simulink model "Esercizio2"  (R2020a)
settings: Solver=VariableStepAuto  StartTime=0.0  StopTime=100  RelTol=1e-3
values from neighbouring files (symbols this model uses):
  D = 0.05    [parameters.m]
  g = 9.8    [parameters.m]
  K = 5    [parameters.m]
  M = 1    [parameters.m]
  x_0 = 10    [parameters.m]
settings Model: Creator=bogda  LastModifiedBy=bogda

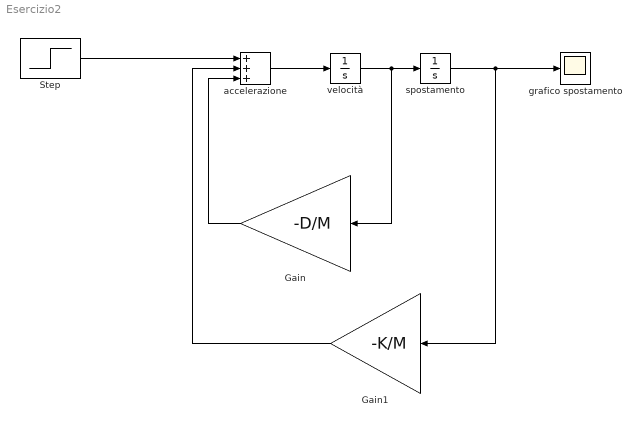
== system Esercizio2 ==
  Gain : Gain  Gain=-D/M
  Gain1 : Gain  Gain=-K/M
  Step : Step  After=g  SampleTime=0
  accelerazione : Sum  Inputs=+++
  grafico spostamento : Scope
  spostamento : Integrator  InitialCondition=x_0
  velocità : Integrator
  wires:
  accelerazione/1 -> velocità/1
  velocità/1 -> Gain/1, spostamento/1
  Step/1 -> accelerazione/1
  spostamento/1 -> Gain1/1, grafico spostamento/1
  Gain/1 -> accelerazione/3
  Gain1/1 -> accelerazione/2
